simulink model "Lab_Modulation_PM"  (R2021b)
settings: Solver=VariableStepAuto  StartTime=0.0  StopTime=10.0  RelTol=1e-3
libraries: dspfdesign x1, commanapbnd3 x1
settings Model: Creator=User  LastModifiedBy=aleksejshevcenko
settings SolverCC: AlgebraicLoopSolver=TrustRegion
settings DataIOCC: ReturnWorkspaceOutputs=off
settings DebuggingCC: SFMachineParentedDataDiag=warning  ArithmeticOperatorsInVariantConditions=warning
settings SFSimCC: SimUseLocalCustomCode=off  CustomCodeUndefinedFunction=UseInterfaceOnly
settings RTWCC: RTWUseLocalCustomCode=off
settings CodeAppCC: StateflowObjectComments=on

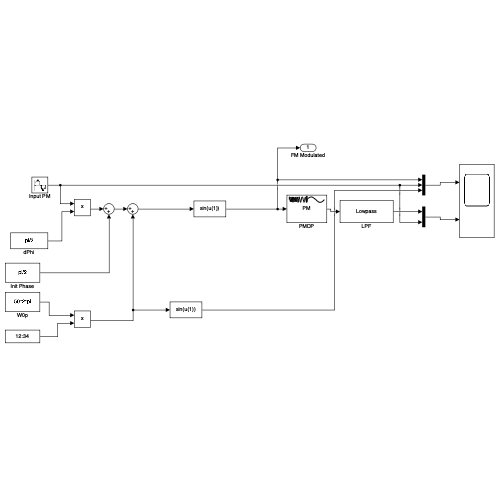
[thumbnail: Simulink's stored preview of the top-level diagram]
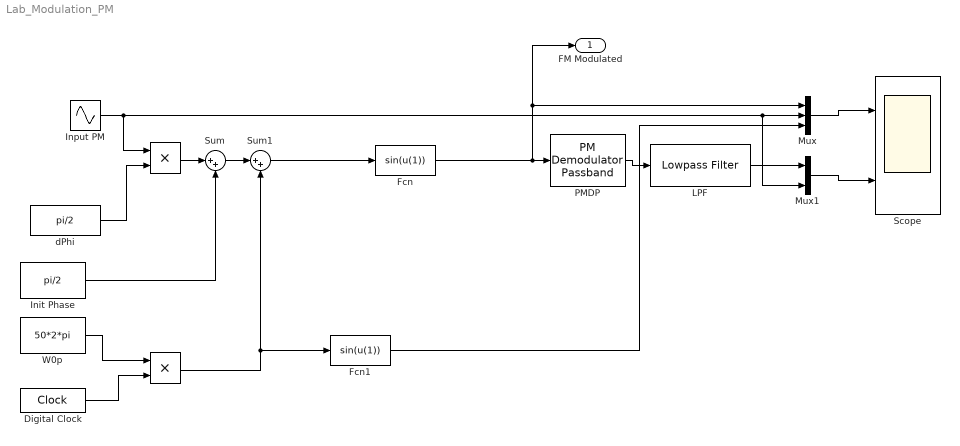
== system Lab_Modulation_PM ==
  " " : Product
  " " : Product
  Digital Clock : DigitalClock  SampleTime=0.0001
  Fcn : Fcn  Expr=sin(u(1))
  Fcn1 : Fcn  Expr=sin(u(1))
  "Init Phase " : Constant  Value=pi/2
  "Input PM " : Sin  Frequency=2*2*pi  SampleTime=0.0001
  "LPF " : dspfdesign/Lowpass Filter  FilterType=FIR  DesignForMinimumOrder=on  FilterOrder=50  PassbandFrequency=0.1  StopbandFrequency=100  PassbandRipple=0.1  StopbandAttenuation=80  InheritSampleRate=on  SampleRate=44100  SimulateUsing=Interpreted execution  roundingMode=Floor  coeffsDataTypeStr=fixdt(1,16)
  Mux : Mux  Inputs=3
  Mux1 : Mux  Inputs=2
  PMDP : commanapbnd3/PM Demodulator Passband  Fc=50  Ph=0  Kc=pi/2  Ho=100
      settings: SourceProductBaseCode=CM
  Scope : Scope  NumInputPorts=2
  Sum : Sum  Inputs=|++
  Sum1 : Sum  Inputs=|++
  "W0p " : Constant  Value=50*2*pi
  dPhi : Constant  Value=pi/2
  FM Modulated : Outport
  wires:
  dPhi/1 -> " "/2
  "Input PM "/1 -> Mux1/2, Mux/2, " "/1
  "Init Phase "/1 -> Sum/2
  " "/1 -> Sum/1
  "LPF "/1 -> Mux1/1
  Mux/1 -> Scope/1
  Mux1/1 -> Scope/2
  Fcn/1 -> PMDP/1, Mux/1, FM Modulated/1
  Digital Clock/1 -> " "/2
  "W0p "/1 -> " "/1
  Sum/1 -> Sum1/1
  " "/1 -> Fcn1/1, Sum1/2
  Fcn1/1 -> Mux/3
  Sum1/1 -> Fcn/1
  PMDP/1 -> "LPF "/1
